simulink model "Alpha_Drone_Model"  (R2020b)
settings: Solver=VariableStepAuto  StartTime=0.0  StopTime=5  RelTol=1e-3
model workspace (MATLAB code in the model file):
  smiData = struct
  smiData.RigidTransform = struct
  smiData.Solid = struct
  smiData.PlanarJoint = struct
  smiData.PlanarJoint.Rz = struct
  smiData.PlanarJoint.Rz.Pos = -154.16759191545947
  smiData.PlanarJoint.Px = struct
  smiData.PlanarJoint.Px.Pos = 0
  smiData.PlanarJoint.Py = struct
  smiData.PlanarJoint.Py.Pos = 0
  smiData.PlanarJoint.ID = '[drone_pillar_test_2-1:-:drone_top_test_3-1]'
  smiData.PrismaticJoint = struct
  smiData.RevoluteJoint = struct
  other statements: smiData.RigidTransform(1).translation =    [0 0 0];; smiData.RigidTransform(1).angle = 3.1415926535897931;; smiData.RigidTransform(1).axis = [1 0 0];; smiData.RigidTransform(1).ID = ['B[drone_base_test_3-1:-:drone_camera_w'                                  'all_test-1]']; smiData.RigidTransform(2).translation =    [88.000000000000028 19.999999999999986 6.00000000000003];; smiData.RigidTransform(2).angle = 2.0943951023931953;; smiData.RigidTransform(2).axis = [0.57735026918962584 0.57735026918962584                                    -0.57735026; smiData.RigidTransform(2).ID = ['F[drone_base_test_3-1:-:drone_camera_w'                                  'all_test-1]']; smiData.RigidTransform(3).translation =    [0 0 0];; smiData.RigidTransform(3).angle = 3.1415926535897931;; smiData.RigidTransform(3).axis = [1 0 0];; smiData.RigidTransform(3).ID = ['B[drone_base_test_3-1:-:drone_camera_w'                                  'all_test-2]'] ... (+385)
undefined symbols (not defined in the file or in its folder): g, R, V1_trim, V3_trim, X, Y, Z
libraries: sm_lib x149, fl_lib x113, nesl_utility x52, ee_lib x16
(part 2 of 5)

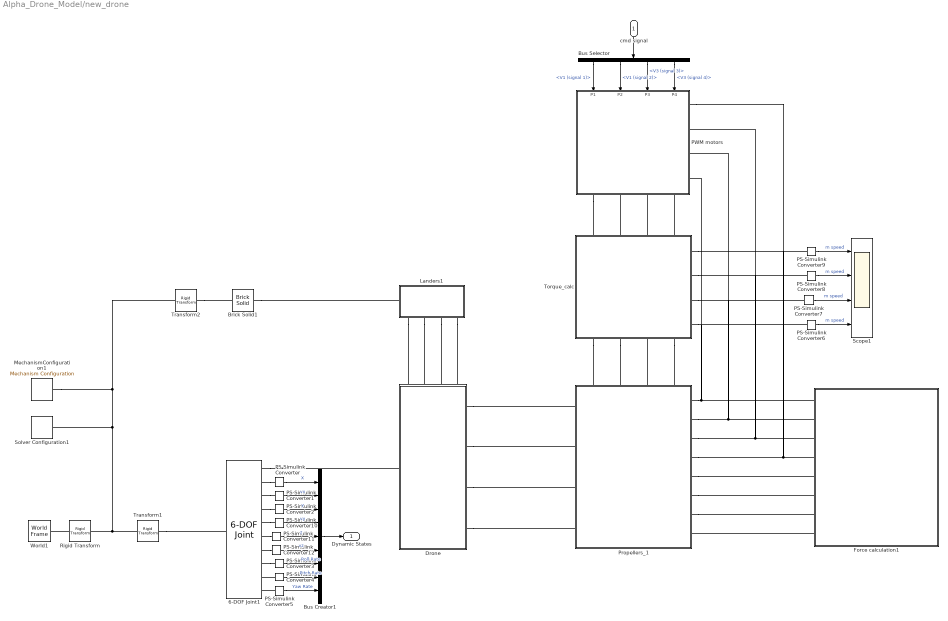
== system Alpha_Drone_Model/new_drone ==
  cmd signal : Inport
  6-DOF Joint1 : sm_lib/Joints/6-DOF Joint  JointMode=Normal  SenseConstraintForce=off  SenseConstraintForceX=off  SenseConstraintForceY=off  SenseConstraintForceZ=off  SenseConstraintTorque=off  SenseConstraintTorqueX=off  SenseConstraintTorqueY=off  SenseConstraintTorqueZ=off  SenseTotalForce=off  SenseTotalForceX=off  SenseTotalForceY=off  SenseTotalForceZ=off  SenseTotalTorque=off  SenseTotalTorqueX=off  SenseTotalTorqueY=off  SenseTotalTorqueZ=off  CompositeWrenchDir=FollowerOnBase  CompositeWrenchFrame=BaseFrame  PxEquilibriumPosition=0  PxEquilibriumPositionUnits=m  PxSpringStiffness=0  PxSpringStiffnessUnits=N/m  PxDampingCoefficient=air_damping  PxDampingCoefficientUnits=N/(m/s)  PxTorqueActuationMode=NoTorque  PxMotionActuationMode=ComputedMotion  PxSensePosition=on  PxSenseVelocity=on  PxSenseAcceleration=off  PxSenseTorqueForce=off  PxSenseLowerLimitTorqueForce=off  PxSenseUpperLimitTorqueForce=off  PxLowerLimitSpecify=off  PxLowerLimitBound=-1  PxLowerLimitBoundUnits=m  PxLowerLimitStiffness=1e6  PxLowerLimitStiffnessUnits=N/m  PxLowerLimitDamping=1e3  PxLowerLimitDampingUnits=N/(m/s)  PxLowerLimitTransitionRegionWidth=1e-4  PxLowerLimitTransitionRegionWidthUnits=m  PxUpperLimitSpecify=off  PxUpperLimitBound=1  PxUpperLimitBoundUnits=m  PxUpperLimitStiffness=1e6  PxUpperLimitStiffnessUnits=N/m  PxUpperLimitDamping=1e3  PxUpperLimitDampingUnits=N/(m/s)  PxUpperLimitTransitionRegionWidth=1e-4  PxUpperLimitTransitionRegionWidthUnits=m  PxPositionTargetSpecify=off  PxPositionTargetPriority=High  PxPositionTargetValue=0  PxPositionTargetValueUnits=m  PxVelocityTargetSpecify=off  PxVelocityTargetPriority=High  PxVelocityTargetValue=0  PxVelocityTargetValueUnits=m/s  PyEquilibriumPosition=0  PyEquilibriumPositionUnits=m  PySpringStiffness=0  PySpringStiffnessUnits=N/m  PyDampingCoefficient=air_damping  PyDampingCoefficientUnits=N/(m/s)  PyTorqueActuationMode=NoTorque  PyMotionActuationMode=ComputedMotion  PySensePosition=on  PySenseVelocity=on  PySenseAcceleration=off  PySenseTorqueForce=off  PySenseLowerLimitTorqueForce=off  PySenseUpperLimitTorqueForce=off  PyLowerLimitSpecify=off  PyLowerLimitBound=0  PyLowerLimitBoundUnits=m  PyLowerLimitStiffness=1e6  PyLowerLimitStiffnessUnits=N/m  PyLowerLimitDamping=1  PyLowerLimitDampingUnits=N/(m/s)  PyLowerLimitTransitionRegionWidth=1e4  PyLowerLimitTransitionRegionWidthUnits=m  PyUpperLimitSpecify=off  PyUpperLimitBound=1  PyUpperLimitBoundUnits=m  PyUpperLimitStiffness=1e6  PyUpperLimitStiffnessUnits=N/m  PyUpperLimitDamping=1e3  PyUpperLimitDampingUnits=N/(m/s)  PyUpperLimitTransitionRegionWidth=1e-4  PyUpperLimitTransitionRegionWidthUnits=m  PyPositionTargetSpecify=off  PyPositionTargetPriority=High  PyPositionTargetValue=0  PyPositionTargetValueUnits=m  PyVelocityTargetSpecify=off  PyVelocityTargetPriority=High  PyVelocityTargetValue=0  PyVelocityTargetValueUnits=m/s  PzEquilibriumPosition=0  PzEquilibriumPositionUnits=m  PzSpringStiffness=0  PzSpringStiffnessUnits=N/m  PzDampingCoefficient=air_damping  PzDampingCoefficientUnits=N/(m/s)  PzTorqueActuationMode=NoTorque  PzMotionActuationMode=ComputedMotion  PzSensePosition=on  PzSenseVelocity=on  PzSenseAcceleration=off  PzSenseTorqueForce=off  PzSenseLowerLimitTorqueForce=off  PzSenseUpperLimitTorqueForce=off  PzLowerLimitSpecify=off  PzLowerLimitBound=-1  PzLowerLimitBoundUnits=m  PzLowerLimitStiffness=1e6  PzLowerLimitStiffnessUnits=N/m  PzLowerLimitDamping=1e3  PzLowerLimitDampingUnits=N/(m/s)  PzLowerLimitTransitionRegionWidth=1e-4  PzLowerLimitTransitionRegionWidthUnits=m  PzUpperLimitSpecify=off  PzUpperLimitBound=1  PzUpperLimitBoundUnits=m  PzUpperLimitStiffness=1e6  PzUpperLimitStiffnessUnits=N/m  PzUpperLimitDamping=1e3  PzUpperLimitDampingUnits=N/(m/s)  PzUpperLimitTransitionRegionWidth=1e-4  PzUpperLimitTransitionRegionWidthUnits=m  PzPositionTargetSpecify=off  PzPositionTargetPriority=High  PzPositionTargetValue=0  PzPositionTargetValueUnits=m  PzVelocityTargetSpecify=off  PzVelocityTargetPriority=High  PzVelocityTargetValue=0  PzVelocityTargetValueUnits=m/s  SphDefPosRotationMethod=None  SphDefPosRotationAngleUnits=deg  SphDefPosRotationStandardAxis=+Z  SphDefPosRotationAngle=0.0  SphDefPosRotationArbitraryAxis=[0 0 1]  SphDefPosFollAlignAxisA=+X  SphDefPosBaseAlignAxisA=+Y  SphDefPosFollAlignAxisB=+Y  SphDefPosBaseAlignAxisB=+Z  SphDefPosRotationSequenceAxes=FollowerAxes  SphDefPosRotationSequence=XYX  SphDefPosRotationSequenceAngles=[0 0 0]  SphDefPosRotationSequenceAnglesUnits=deg  SphDefPosRotationMatrix=[1 0 0; 0 1 0; 0 0 1]  SphEqPosRotationMethod=None  SphEqPosRotationAngleUnits=deg  SphEqPosRotationStandardAxis=+Z  SphEqPosRotationAngle=0.0  SphEqPosRotationArbitraryAxis=[0 0 1]  SphEqPosFollAlignAxisA=+X  SphEqPosBaseAlignAxisA=+Y  SphEqPosFollAlignAxisB=+Y  SphEqPosBaseAlignAxisB=+Z  SphEqPosRotationSequenceAxes=FollowerAxes  SphEqPosRotationSequence=XYX  SphEqPosRotationSequenceAngles=[0 0 0]  SphEqPosRotationSequenceAnglesUnits=deg  SphEqPosRotationMatrix=[1 0 0; 0 1 0; 0 0 1]  SphSpringStiffness=0  SphSpringStiffnessUnits=N*m/deg  SphDampingCoefficient=air_damping  SphDampingCoefficientUnits=N*m/(deg/s)  SphActuateTorqueX=off  SphActuateTorqueY=off  SphActuateTorqueZ=off  SphActuateTorque=off  SphTorqueActuationMode=NoTorque  SphMotionActuationMode=ComputedMotion  SphActuationFrame=BaseFrame  SphSensePosition=off  SphSenseVelocityX=on  SphSenseVelocityY=on  SphSenseVelocityZ=on  SphSenseVelocity=off  SphSenseAccelerationX=off  SphSenseAccelerationY=off  SphSenseAccelerationZ=off  SphSenseAcceleration=off  SphSenseTorqueX=off  SphSenseTorqueY=off  SphSenseTorqueZ=off  SphSenseTorqueForce=off  SphSenseLowerLimitTorqueMag=off  SphSenseUpperLimitTorqueMag=off  SphSensingFrame=BaseFrame  SphLowerLimitSpecify=off  SphLowerLimitBound=15  SphLowerLimitBoundUnits=deg  SphLowerLimitStiffness=1e4  SphLowerLimitStiffnessUnits=N*m/deg  SphLowerLimitDamping=10  SphLowerLimitDampingUnits=N*m/(deg/s)  SphLowerLimitTransitionRegionWidth=0.1  SphLowerLimitTransitionRegionWidthUnits=deg  SphUpperLimitSpecify=off  SphUpperLimitBound=45  SphUpperLimitBoundUnits=deg  SphUpperLimitStiffness=1e4  SphUpperLimitStiffnessUnits=N*m/deg  SphUpperLimitDamping=10  SphUpperLimitDampingUnits=N*m/(deg/s)  SphUpperLimitTransitionRegionWidth=0.1  SphUpperLimitTransitionRegionWidthUnits=deg  SphPositionTargetRotationMethod=AlignedAxes  SphPositionTargetRotationAngleUnits=deg  SphPositionTargetRotationStandardAxis=+Z  SphPositionTargetRotationAngle=0.0  SphPositionTargetRotationArbitraryAxis=[0 0 1]  SphPositionTargetFollAlignAxisA=+X  SphPositionTargetBaseAlignAxisA=+X  SphPositionTargetFollAlignAxisB=+Y  SphPositionTargetBaseAlignAxisB=+Y  SphPositionTargetRotationSequenceAxes=FollowerAxes  SphPositionTargetRotationSequence=XYX  SphPositionTargetRotationSequenceAngles=[0 0 0]  SphPositionTargetRotationSequenceAnglesUnits=deg  SphPositionTargetRotationMatrix=[1 0 0; 0 1 0; 0 0 1]  SphPositionTargetSpecify=off  SphPositionTargetPriority=High  SphVelocityTargetValue=[0 0 0]  SphVelocityTargetValueUnits=deg/s  SphVelocityTargetSpecify=off  SphVelocityTargetPriority=High  SphVelocityTargetInFollowerFrame=on
  Brick Solid1 : sm_lib/Body Elements/Brick Solid  GraphicAmbientColor=[0.15 0.15 0.15 1.0]  BasedOnType=Density  BrickDimensions=[1 1 0.1]  BrickDimensionUnits=m  CenterOfMass=[0 0 0]  CenterOfMassUnits=m  GraphicDiffuseColor=[0.0 0.6 0.2]  Density=1000  DensityUnits=kg/m^3  DoExposeReferenceFrame=on  GraphicEmissiveColor=[0.0 0.0 0.0 1.0]  ExportEntireGeometry=on  SerializedFrames=<Frames/>  MarkerShape=Sphere  MarkerSize=10  GraphicType=FromGeometry  InertiaType=CalculateFromGeometry  Mass=1  MassUnits=kg  MomentsOfInertia=[1 1 1]  MomentsOfInertiaUnits=kg*m^2  GraphicOpacity=1.0  ProductsOfInertia=[0 0 0]  ProductsOfInertiaUnits=kg*m^2  GraphicShininess=75  GraphicSpecularColor=[0.5 0.5 0.5 1.0]  GraphicVisPropType=SimpleVisualProperties
  Bus Creator1 : BusCreator  Inputs=9
  Bus Selector : BusSelector  OutputSignals=V1 (signal 1),V1 (signal 2),V3 (signal 3),V3 (signal 4)
  Drone : Subsystem
      settings: PortSchema="{\"entries\":[{\"content\":{\"sides\":[{\"content\":{\"connectorIds\":[\"LConn1\"]},\"type\":\"ConnectorPlacement.EquallySpacedRectSide\",\"uuid\":\"2ddff43e-b9b9-4f8b-b52c-32ef76abc7f2\"},{\"content\":{\"connectorIds\":[\"RConn1\",\"RConn2\",\"RConn3\",\"RConn4\"],\"side\":\"RIGHT\"},\"type\":\"ConnectorPlacement.EquallySpacedRectSide\",\"uuid\":\"84cdcda4-30ad-4435-863c-4e05e54e1cee\"},{\"content\":{\"connectorIds\":[\"LConn2\",\"LConn3\",\"LConn4\",\"LConn5\"],\"side\":\"TOP\"},\"type\":\"ConnectorPlacement.EquallySpacedRectSide\",\"uuid\":\"12774c4c-303b-498f-8577-32bcc0aee797\"},{\"content\":{\"connectorIds\":[],\"side\":\"HIDDEN\"},\"type\":\"ConnectorPlacement.EquallySpacedRectSide\",\"uuid\":\"2c89ce61-ca11-462f-b06b-bd195c97151b\"}]},\"type\":\"ConnectorPlacement.EquallySpacedConnector\",\"uuid\":\"ae66c99c-2a8a-4601-9c2b-027ea84a534a\"}],\"packageUris\":[\"http://schema.mathworks.com/mf0/Connector/R2020b\"],\"version\":\"1.0\"}"
  Force calculation1 : Subsystem
  Landers1 : Subsystem
      settings: PortSchema="{\"entries\":[{\"content\":{\"sides\":[{\"content\":{\"connectorIds\":[]},\"type\":\"ConnectorPlacement.EquallySpacedRectSide\",\"uuid\":\"29ed25fe-b3f0-40d8-8e38-dad31f47c1c2\"},{\"content\":{\"connectorIds\":[\"RConn1\"],\"side\":\"RIGHT\"},\"type\":\"ConnectorPlacement.EquallySpacedRectSide\",\"uuid\":\"a44326be-c514-4699-a20f-f031abb9163a\"},{\"content\":{\"connectorIds\":[\"LConn1\",\"LConn2\",\"LConn3\",\"LConn4\"],\"side\":\"TOP\"},\"type\":\"ConnectorPlacement.EquallySpacedRectSide\",\"uuid\":\"e989b3f4-324c-4714-b27e-b8d073d4c35f\"},{\"content\":{\"connectorIds\":[],\"side\":\"HIDDEN\"},\"type\":\"ConnectorPlacement.EquallySpacedRectSide\",\"uuid\":\"003ab62d-37b6-4b48-957b-1f2b95d598b0\"}]},\"type\":\"ConnectorPlacement.EquallySpacedConnector\",\"uuid\":\"ee59c263-ccee-4526-9944-481878d464b1\"}],\"packageUris\":[\"http://schema.mathworks.com/mf0/Connector/R2020b\"],\"version\":\"1.0\"}"
  MechanismConfiguration1 : sm_lib/Utilities/Mechanism Configuration  UniformGravity=Constant  GravityVector=[0 0 g]  GravityVectorUnits=m/s^2  GravityUnits=m/s^2  LinearizationDelta=0.001  JointModeTransitionNonlinearIterations=2
  PS-Simulink Converter{,1..5,10..12} (9 alike) : nesl_utility/PS-Simulink Converter  PhysicalDomain=network_engine_domain  SubClassName=ps_output  LeftPortType=input  RightPortType=output  PseudoPeriodic=off  Frequencies=[]  Unit=inherit  AffineConversion=off
  PS-Simulink Converter{6..9} (4 alike) : nesl_utility/PS-Simulink Converter  PhysicalDomain=network_engine_domain  SubClassName=ps_output  LeftPortType=input  RightPortType=output  PseudoPeriodic=off  Frequencies=[]  Unit=rpm  AffineConversion=off
  PWM motors : Subsystem
      settings: PortSchema="{\"entries\":[{\"content\":{\"sides\":[{\"content\":{\"connectorIds\":[\"In1\",\"In2\",\"In3\",\"In4\"]},\"type\":\"ConnectorPlacement.EquallySpacedRectSide\",\"uuid\":\"0aa47eaa-b314-49af-ba20-9f866096b1c7\"},{\"content\":{\"connectorIds\":[\"RConn1\",\"RConn2\",\"RConn3\",\"RConn4\"],\"side\":\"RIGHT\"},\"type\":\"ConnectorPlacement.EquallySpacedRectSide\",\"uuid\":\"be00fcf1-f0c0-4679-a976-81a7113ef2f3\"},{\"content\":{\"connectorIds\":[],\"side\":\"TOP\"},\"type\":\"ConnectorPlacement.EquallySpacedRectSide\",\"uuid\":\"744c4fca-265d-4f23-9ed8-a5ce9174507b\"},{\"content\":{\"connectorIds\":[\"RConn5\",\"RConn6\",\"RConn7\",\"RConn8\"],\"side\":\"BOTTOM\"},\"type\":\"ConnectorPlacement.EquallySpacedRectSide\",\"uuid\":\"b07c2b3a-f3e9-41e5-9730-85c6be094db7\"},{\"content\":{\"connectorIds\":[],\"side\":\"HIDDEN\"},\"type\":\"ConnectorPlacement.EquallySpacedRectSide\",\"uuid\":\"b49dea78-7ad3-4d52-b3a6-72cc1bd77d5e\"}]},\"type\":\"ConnectorPlacement.EquallySpacedConnector\",\"uuid\":\"57264236-7f66-4868-aca9-e0c74f83ab49\"}],\"packageUris\":[\"http://schema.mathworks.com/mf0/Connector/R2020b\"],\"version\":\"1.0\"}"
  Propellers_1 : Subsystem
      settings: PortSchema="{\"entries\":[{\"content\":{\"sides\":[{\"content\":{\"connectorIds\":[\"LConn1\",\"LConn2\",\"LConn3\",\"LConn4\"]},\"type\":\"ConnectorPlacement.EquallySpacedRectSide\",\"uuid\":\"b250e274-2fd6-45d7-b915-b466c5f9d255\"},{\"content\":{\"connectorIds\":[\"RConn1\",\"RConn2\",\"RConn3\",\"RConn4\",\"RConn5\",\"RConn6\",\"RConn7\",\"RConn8\"],\"side\":\"RIGHT\"},\"type\":\"ConnectorPlacement.EquallySpacedRectSide\",\"uuid\":\"c76b79cf-ecc8-43fa-b8c8-dc402773d11f\"},{\"content\":{\"connectorIds\":[\"LConn5\",\"LConn6\",\"LConn7\",\"LConn8\"],\"side\":\"TOP\"},\"type\":\"ConnectorPlacement.EquallySpacedRectSide\",\"uuid\":\"3950bb13-7450-4adc-a891-c6053fed2cc6\"},{\"content\":{\"connectorIds\":[],\"side\":\"HIDDEN\"},\"type\":\"ConnectorPlacement.EquallySpacedRectSide\",\"uuid\":\"c1ecd3aa-adb0-4a11-9d33-da842965230c\"}]},\"type\":\"ConnectorPlacement.EquallySpacedConnector\",\"uuid\":\"e31fcf3f-0f5a-48dc-bc44-b2ff7b3cb046\"}],\"packageUris\":[\"http://schema.mathworks.com/mf0/Connector/R2020b\"],\"version\":\"1.0\"}"
  Rigid Transform : sm_lib/Frames and Transforms/Rigid Transform  TranslationMethod=None  TranslationStandardOffset=0  TranslationLengthUnit=m  TranslationStandardAxis=+Z  TranslationCartesianOffset=[0 0 0]  TranslationROffset=0  TranslationROffsetUnits=m  TranslationZOffset=0  TranslationZOffsetUnits=m  TranslationThetaOffset=0  TranslationThetaOffsetUnits=deg  RotationMethod=StandardAxis  RotationAngleUnits=deg  RotationStandardAxis=+X  RotationAngle=180  RotationArbitraryAxis=[0 0 1]  FollAlignAxisA=+X  BaseAlignAxisA=+Y  FollAlignAxisB=+Y  BaseAlignAxisB=+Z  RotationSequenceAxes=FollowerAxes  RotationSequence=XYX  RotationSequenceAngles=[0 0 0]  RotationSequenceAnglesUnits=deg  RotationMatrix=[1 0 0; 0 1 0; 0 0 1]
  Scope1 : Scope  NumInputPorts=4
  Solver Configuration1 : nesl_utility/Solver Configuration  PhysicalDomain=network_engine_domain  SubClassName=solver  LeftPortType=input  RightPortType=generic  Tones=[]  Harmonics=[]  SimulateNoise=off  Profile=off  UseLocalSampling=off  EnableSwitchedLinearOptims=on  FrequencyDomain=off  UseCCode=off  RelTol=0.001  AbsTol=1e-06  MinStep=1e-09  ToWorkspace=off  RevertToSquareIcSolve=off  NumHomotopyIterations=100  PhasorMode=off  PhasorModeNumHarmonics=1  DoDC=off  ResidualTolerance=1e-09  UseLocalSolver=off  LocalSolverChoice=NE_BACKWARD_EULER_ADVANCER  LocalSolverSampleTime=0.001  DoFixedCost=off  MaxNonlinIter=3  MaxModeIter=2  ComputeImpulses=off  ImpulseIterations=2  LinearAlgebra=auto  EquationFormulation=NE_TIME_EF  DelaysMemoryBudget=1024  AutomaticFiltering=on  FilteringTimeConstant=0.001  PartitionStorageMethod=AS_NEEDED  PartitionMemoryBudget=1024  PartitionMethod=ROBUST
  Torque_calc : Subsystem
      settings: PortSchema="{\"entries\":[{\"content\":{\"sides\":[{\"content\":{\"connectorIds\":[]},\"type\":\"ConnectorPlacement.EquallySpacedRectSide\",\"uuid\":\"eea3dfa4-6c4f-447d-9f2a-f18a83183d98\"},{\"content\":{\"connectorIds\":[\"RConn1\",\"RConn2\",\"RConn3\",\"RConn4\"],\"side\":\"RIGHT\"},\"type\":\"ConnectorPlacement.EquallySpacedRectSide\",\"uuid\":\"c604e34d-0590-453f-bf6c-420895a89f4d\"},{\"content\":{\"connectorIds\":[\"LConn1\",\"LConn2\",\"LConn3\",\"LConn4\"],\"side\":\"TOP\"},\"type\":\"ConnectorPlacement.EquallySpacedRectSide\",\"uuid\":\"50bcecdb-52f6-4b25-bece-8e6a846b7dd0\"},{\"content\":{\"connectorIds\":[\"RConn5\",\"RConn6\",\"RConn7\",\"RConn8\"],\"side\":\"BOTTOM\"},\"type\":\"ConnectorPlacement.EquallySpacedRectSide\",\"uuid\":\"c913db90-ccc2-4f4f-a5da-6c9411a23c28\"},{\"content\":{\"connectorIds\":[],\"side\":\"HIDDEN\"},\"type\":\"ConnectorPlacement.EquallySpacedRectSide\",\"uuid\":\"0f1aeb6e-b451-4600-ac15-69882e2b4329\"}]},\"type\":\"ConnectorPlacement.EquallySpacedConnector\",\"uuid\":\"f9536a7f-9aaa-4e3e-af48-cb10a5d231a4\"}],\"packageUris\":[\"http://schema.mathworks.com/mf0/Connector/R2020b\"],\"version\":\"1.0\"}"
  Transform1 : sm_lib/Frames and Transforms/Rigid Transform  TranslationMethod=StandardAxis  TranslationStandardOffset=0.1  TranslationLengthUnit=m  TranslationStandardAxis=-Z  TranslationCartesianOffset=smiData.RigidTransform(63).translation  TranslationROffset=0  TranslationROffsetUnits=m  TranslationZOffset=0  TranslationZOffsetUnits=m  TranslationThetaOffset=0  TranslationThetaOffsetUnits=deg  RotationMethod=None  RotationAngleUnits=rad  RotationStandardAxis=+Z  RotationAngle=smiData.RigidTransform(63).angle  RotationArbitraryAxis=smiData.RigidTransform(63).axis  FollAlignAxisA=+X  BaseAlignAxisA=+Y  FollAlignAxisB=+Y  BaseAlignAxisB=+Z  RotationSequenceAxes=FollowerAxes  RotationSequence=XYX  RotationSequenceAngles=[0 0 0]  RotationSequenceAnglesUnits=deg  RotationMatrix=[1 0 0; 0 1 0; 0 0 1]
  Transform2 : sm_lib/Frames and Transforms/Rigid Transform  TranslationMethod=StandardAxis  TranslationStandardOffset=0.05  TranslationLengthUnit=m  TranslationStandardAxis=+Z  TranslationCartesianOffset=smiData.RigidTransform(63).translation  TranslationROffset=0  TranslationROffsetUnits=m  TranslationZOffset=0  TranslationZOffsetUnits=m  TranslationThetaOffset=0  TranslationThetaOffsetUnits=deg  RotationMethod=None  RotationAngleUnits=deg  RotationStandardAxis=+X  RotationAngle=180  RotationArbitraryAxis=smiData.RigidTransform(63).axis  FollAlignAxisA=+X  BaseAlignAxisA=+Y  FollAlignAxisB=+Y  BaseAlignAxisB=+Z  RotationSequenceAxes=FollowerAxes  RotationSequence=XYX  RotationSequenceAngles=[0 0 0]  RotationSequenceAnglesUnits=deg  RotationMatrix=[1 0 0; 0 1 0; 0 0 1]
  World1 : sm_lib/Frames and Transforms/World Frame
  Dynamic States : Outport
  wires:
  PS-Simulink Converter4/1 -> Bus Creator1/8  "Pitch Rate"
  PS-Simulink Converter/1 -> Bus Creator1/1  "X"
  PS-Simulink Converter3/1 -> Bus Creator1/7  "Roll Rate"
  PS-Simulink Converter5/1 -> Bus Creator1/9  "Yaw Rate"
  Bus Creator1/1 -> Dynamic States/1
  PS-Simulink Converter6/1 -> Scope1/4  "m speed"
  PS-Simulink Converter7/1 -> Scope1/3  "m speed"
  PS-Simulink Converter8/1 -> Scope1/2  "m speed"
  PS-Simulink Converter9/1 -> Scope1/1  "m speed"
  cmd signal/1 -> Bus Selector/1
  PS-Simulink Converter2/1 -> Bus Creator1/3  "y"
  PS-Simulink Converter11/1 -> Bus Creator1/5  "z"
  PS-Simulink Converter1/1 -> Bus Creator1/2  "vx"
  PS-Simulink Converter10/1 -> Bus Creator1/4  "vy"
  PS-Simulink Converter12/1 -> Bus Creator1/6  "vz"
  Bus Selector/1 -> PWM motors/1(P1)  "<V1 (signal 1)>"
  Bus Selector/2 -> PWM motors/2(P2)  "<V1 (signal 2)>"
  Bus Selector/3 -> PWM motors/3(P3)  "<V3 (signal 3)>"
  Bus Selector/4 -> PWM motors/4(P4)  "<V3 (signal 4)>"
  connections:
  Propellers_1/RConn1 -- PS-Simulink Converter6/LConn1 -- Torque_calc/RConn4 -- PWM motors/RConn8 -- Force calculation1/LConn1
  Landers1/LConn1 -- Drone/LConn5
  Propellers_1/RConn7 -- Force calculation1/LConn7
  Propellers_1/RConn4 -- PWM motors/RConn5 -- PS-Simulink Converter9/LConn1 -- Torque_calc/RConn1 -- Force calculation1/LConn4
  Landers1/LConn2 -- Drone/LConn4
  Drone/RConn1 -- Propellers_1/LConn1
  Landers1/LConn4 -- Drone/LConn2
  Propellers_1/RConn6 -- Force calculation1/LConn6
  Propellers_1/RConn5 -- Force calculation1/LConn5
  Drone/RConn4 -- Propellers_1/LConn4
  Landers1/LConn3 -- Drone/LConn3
  Drone/RConn3 -- Propellers_1/LConn3
  Force calculation1/LConn8 -- Propellers_1/RConn8
  Drone/RConn2 -- Propellers_1/LConn2
  Propellers_1/RConn3 -- PS-Simulink Converter8/LConn1 -- Torque_calc/RConn2 -- PWM motors/RConn6 -- Force calculation1/LConn3
  Propellers_1/RConn2 -- Force calculation1/LConn2 -- PWM motors/RConn7 -- PS-Simulink Converter7/LConn1 -- Torque_calc/RConn3
  PWM motors/RConn1 -- Torque_calc/LConn1
  Torque_calc/LConn3 -- PWM motors/RConn3
  Torque_calc/LConn2 -- PWM motors/RConn2
  Torque_calc/LConn4 -- PWM motors/RConn4
  Torque_calc/RConn5 -- Propellers_1/LConn5
  Propellers_1/LConn7 -- Torque_calc/RConn7
  Torque_calc/RConn6 -- Propellers_1/LConn6
  Torque_calc/RConn8 -- Propellers_1/LConn8
  Transform2/RConn1 -- Brick Solid1/RConn1
  Transform1/LConn1 -- Rigid Transform/RConn1 -- Transform2/LConn1 -- MechanismConfiguration1/RConn1 -- Solver Configuration1/RConn1
  Brick Solid1/LConn1 -- Landers1/RConn1
  Rigid Transform/LConn1 -- World1/RConn1
  6-DOF Joint1/RConn8 -- PS-Simulink Converter3/LConn1
  PS-Simulink Converter4/LConn1 -- 6-DOF Joint1/RConn9
  PS-Simulink Converter5/LConn1 -- 6-DOF Joint1/RConn10
  6-DOF Joint1/RConn2 -- PS-Simulink Converter/LConn1
  6-DOF Joint1/RConn3 -- PS-Simulink Converter1/LConn1
  6-DOF Joint1/RConn4 -- PS-Simulink Converter2/LConn1
  6-DOF Joint1/RConn5 -- PS-Simulink Converter10/LConn1
  6-DOF Joint1/RConn6 -- PS-Simulink Converter11/LConn1
  6-DOF Joint1/RConn7 -- PS-Simulink Converter12/LConn1
  Transform1/RConn1 -- 6-DOF Joint1/LConn1
  6-DOF Joint1/RConn1 -- Drone/LConn1

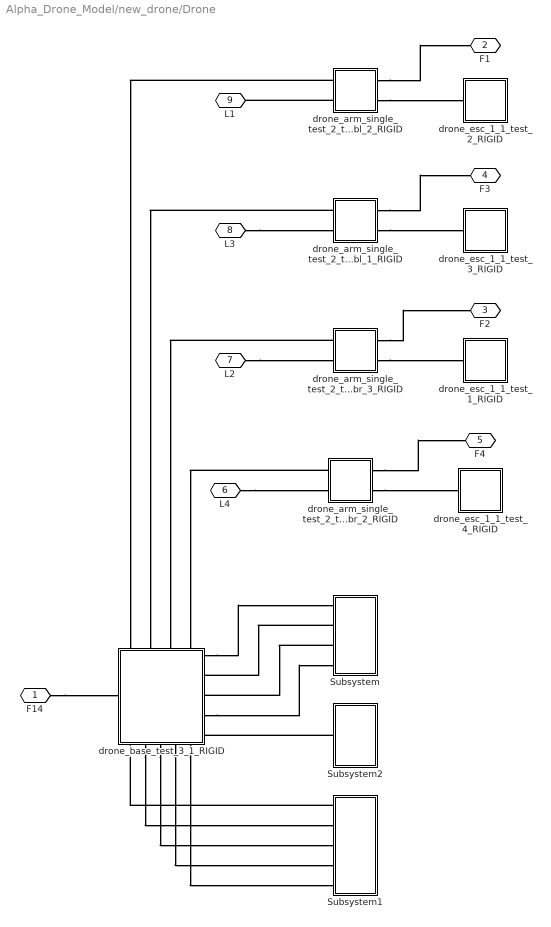
== system Alpha_Drone_Model/new_drone/Drone ==
  Subsystem : Subsystem
  Subsystem1 : Subsystem
  Subsystem2 : Subsystem
  drone_arm_single_test_2_tl_br_2_RIGID : Subsystem
  drone_arm_single_test_2_tl_br_3_RIGID : Subsystem
  drone_arm_single_test_2_tr_bl_1_RIGID : Subsystem
  drone_arm_single_test_2_tr_bl_2_RIGID : Subsystem
  drone_base_test_3_1_RIGID : Subsystem
      settings: PortSchema="{\"entries\":[{\"content\":{\"sides\":[{\"content\":{\"connectorIds\":[\"LConn1\"]},\"type\":\"ConnectorPlacement.EquallySpacedRectSide\",\"uuid\":\"3979f689-f2e7-42c3-80af-f898cffc6627\"},{\"content\":{\"connectorIds\":[\"RConn1\",\"RConn2\",\"RConn3\",\"RConn4\",\"RConn5\"],\"side\":\"RIGHT\"},\"type\":\"ConnectorPlacement.EquallySpacedRectSide\",\"uuid\":\"d5df15a2-0509-4ce9-a78a-c9b521a28f2c\"},{\"content\":{\"connectorIds\":[\"LConn2\",\"LConn3\",\"LConn4\",\"LConn5\"],\"side\":\"TOP\"},\"type\":\"ConnectorPlacement.EquallySpacedRectSide\",\"uuid\":\"a062ce0d-f5a1-4bb9-aa4f-f81fc5481e55\"},{\"content\":{\"connectorIds\":[\"RConn6\",\"RConn7\",\"RConn8\",\"RConn9\",\"RConn10\"],\"side\":\"BOTTOM\"},\"type\":\"ConnectorPlacement.EquallySpacedRectSide\",\"uuid\":\"9e3fb357-542a-46da-bf60-66e0768f6863\"},{\"content\":{\"connectorIds\":[],\"side\":\"HIDDEN\"},\"type\":\"ConnectorPlacement.EquallySpacedRectSide\",\"uuid\":\"788c0c2e-9632-4521-be72-6a644cdbf0ea\"}]},\"type\":\"ConnectorPlacement.EquallySpacedConnector\",\"uuid\":\"1be13487-ca5d-4f55-9a83-a878693f11fe\"}],\"packageUris\":[\"http://schema.mathworks.com/mf0/Connector/R2020b\"],\"version\":\"1.0\"}"
  drone_esc_1_1_test_1_RIGID : Subsystem
  drone_esc_1_1_test_2_RIGID : Subsystem
  drone_esc_1_1_test_3_RIGID : Subsystem
  drone_esc_1_1_test_4_RIGID : Subsystem
  F14 : PMIOPort  Side=Left
  F1 : PMIOPort  Port=2  Side=Right
  F2 : PMIOPort  Port=3  Side=Right
  F3 : PMIOPort  Port=4  Side=Right
  F4 : PMIOPort  Port=5  Side=Right
  L4 : PMIOPort  Port=6  Side=Left
  L2 : PMIOPort  Port=7  Side=Left
  L3 : PMIOPort  Port=8  Side=Left
  L1 : PMIOPort  Port=9  Side=Left
  connections:
  drone_arm_single_test_2_tr_bl_1_RIGID/RConn2 -- drone_esc_1_1_test_3_RIGID/LConn1
  drone_arm_single_test_2_tr_bl_2_RIGID/LConn1 -- drone_base_test_3_1_RIGID/LConn2
  drone_arm_single_test_2_tr_bl_1_RIGID/RConn1 -- F3/RConn1
  drone_arm_single_test_2_tl_br_2_RIGID/RConn2 -- drone_esc_1_1_test_4_RIGID/LConn1
  drone_arm_single_test_2_tl_br_2_RIGID/RConn1 -- F4/RConn1
  drone_arm_single_test_2_tl_br_3_RIGID/RConn2 -- drone_esc_1_1_test_1_RIGID/LConn1
  drone_arm_single_test_2_tr_bl_2_RIGID/RConn2 -- drone_esc_1_1_test_2_RIGID/LConn1
  F14/RConn1 -- drone_base_test_3_1_RIGID/LConn1
  drone_arm_single_test_2_tr_bl_1_RIGID/LConn1 -- drone_base_test_3_1_RIGID/LConn3
  drone_arm_single_test_2_tl_br_2_RIGID/LConn1 -- drone_base_test_3_1_RIGID/LConn5
  drone_arm_single_test_2_tl_br_3_RIGID/LConn1 -- drone_base_test_3_1_RIGID/LConn4
  drone_arm_single_test_2_tr_bl_2_RIGID/RConn1 -- F1/RConn1
  drone_arm_single_test_2_tl_br_3_RIGID/RConn1 -- F2/RConn1
  drone_base_test_3_1_RIGID/RConn1 -- Subsystem/LConn1
  Subsystem/LConn2 -- drone_base_test_3_1_RIGID/RConn2
  Subsystem/LConn3 -- drone_base_test_3_1_RIGID/RConn3
  drone_base_test_3_1_RIGID/RConn4 -- Subsystem/LConn4
  drone_arm_single_test_2_tr_bl_2_RIGID/LConn2 -- L1/RConn1
  L3/RConn1 -- drone_arm_single_test_2_tr_bl_1_RIGID/LConn2
  L2/RConn1 -- drone_arm_single_test_2_tl_br_3_RIGID/LConn2
  L4/RConn1 -- drone_arm_single_test_2_tl_br_2_RIGID/LConn2
  Subsystem1/LConn1 -- drone_base_test_3_1_RIGID/RConn6
  drone_base_test_3_1_RIGID/RConn7 -- Subsystem1/LConn2
  drone_base_test_3_1_RIGID/RConn8 -- Subsystem1/LConn3
  drone_base_test_3_1_RIGID/RConn9 -- Subsystem1/LConn4
  drone_base_test_3_1_RIGID/RConn10 -- Subsystem1/LConn5
  Subsystem2/LConn1 -- drone_base_test_3_1_RIGID/RConn5

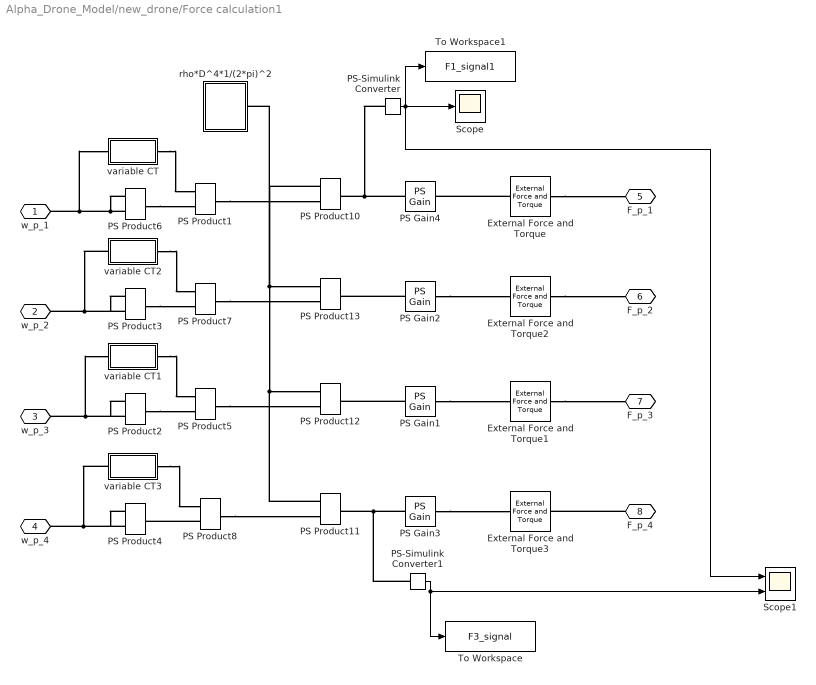
== system Alpha_Drone_Model/new_drone/Force calculation1 ==
  External Force and Torque{,1..3} (4 alike) : sm_lib/Forces and Torques/External Force and Torque  ForceResolutionFrame=AttachedFrame  EnableForceX=off  EnableForceY=off  EnableForceZ=on  EnableForce=off  TorqueResolutionFrame=AttachedFrame  EnableTorqueX=off  EnableTorqueY=off  EnableTorqueZ=off  EnableTorque=off
  PS Gain1 : fl_lib/Physical Signals/Functions/PS Gain  gain=1
  PS Gain2 : fl_lib/Physical Signals/Functions/PS Gain  gain=-1
  PS Gain3 : fl_lib/Physical Signals/Functions/PS Gain  gain=-1
  PS Gain4 : fl_lib/Physical Signals/Functions/PS Gain  gain=1
  PS Product{1..8,10..13} (12 alike) : fl_lib/Physical Signals/Functions/PS Product
  PS-Simulink Converter : nesl_utility/PS-Simulink Converter  PhysicalDomain=network_engine_domain  SubClassName=ps_output  LeftPortType=input  RightPortType=output  PseudoPeriodic=off  Frequencies=[]  Unit=inherit  AffineConversion=off
  PS-Simulink Converter1 : nesl_utility/PS-Simulink Converter  PhysicalDomain=network_engine_domain  SubClassName=ps_output  LeftPortType=input  RightPortType=output  PseudoPeriodic=off  Frequencies=[]  Unit=inherit  AffineConversion=off
  Scope : Scope
  Scope1 : Scope  NumInputPorts=2
  To Workspace : ToWorkspace  VariableName=F3_signal  SampleTime=-1
  To Workspace1 : ToWorkspace  VariableName=F1_signal1  SampleTime=-1
  rho*D^4*1/(2*pi)^2 : Subsystem
  variable CT : Subsystem
  variable CT1 : Subsystem
  variable CT2 : Subsystem
  variable CT3 : Subsystem
  w_p_1 : PMIOPort  Side=Left
  w_p_2 : PMIOPort  Port=2  Side=Left
  w_p_3 : PMIOPort  Port=3  Side=Left
  w_p_4 : PMIOPort  Port=4  Side=Left
  F_p_1 : PMIOPort  Port=5  Side=Left
  F_p_2 : PMIOPort  Port=6  Side=Left
  F_p_3 : PMIOPort  Port=7  Side=Left
  F_p_4 : PMIOPort  Port=8  Side=Left
  wires:
  PS-Simulink Converter/1 -> To Workspace1/1, Scope1/1, Scope/1
  PS-Simulink Converter1/1 -> To Workspace/1, Scope1/2
  connections:
  External Force and Torque2/RConn1 -- F_p_2/RConn1
  External Force and Torque/RConn1 -- F_p_1/RConn1
  External Force and Torque1/RConn1 -- F_p_3/RConn1
  F_p_4/RConn1 -- External Force and Torque3/RConn1
  PS Product6/LConn2 -- PS Product6/LConn1 -- w_p_1/RConn1 -- variable CT/LConn1
  External Force and Torque/LConn1 -- PS Gain4/RConn1
  PS Gain1/RConn1 -- External Force and Torque1/LConn1
  PS Gain2/RConn1 -- External Force and Torque2/LConn1
  PS Gain3/RConn1 -- External Force and Torque3/LConn1
  PS-Simulink Converter/LConn1 -- PS Product10/RConn1 -- PS Gain4/LConn1
  PS-Simulink Converter1/LConn1 -- PS Product11/RConn1 -- PS Gain3/LConn1
  PS Product2/LConn2 -- PS Product2/LConn1 -- variable CT1/LConn1 -- w_p_3/RConn1
  PS Product3/LConn2 -- PS Product3/LConn1 -- variable CT2/LConn1 -- w_p_2/RConn1
  PS Product4/LConn2 -- PS Product4/LConn1 -- variable CT3/LConn1 -- w_p_4/RConn1
  variable CT/RConn1 -- PS Product1/LConn1
  rho*D^4*1/(2*pi)^2/RConn1 -- PS Product10/LConn1 -- PS Product11/LConn1 -- PS Product12/LConn1 -- PS Product13/LConn1
  PS Product6/RConn1 -- PS Product1/LConn2
  PS Product1/RConn1 -- PS Product10/LConn2
  variable CT1/RConn1 -- PS Product5/LConn1
  PS Product2/RConn1 -- PS Product5/LConn2
  PS Product5/RConn1 -- PS Product12/LConn2
  PS Product3/RConn1 -- PS Product7/LConn2
  variable CT2/RConn1 -- PS Product7/LConn1
  PS Product7/RConn1 -- PS Product13/LConn2
  PS Product8/RConn1 -- PS Product11/LConn2
  PS Product8/LConn2 -- PS Product4/RConn1
  variable CT3/RConn1 -- PS Product8/LConn1
  PS Gain2/LConn1 -- PS Product13/RConn1
  PS Gain1/LConn1 -- PS Product12/RConn1

== system Alpha_Drone_Model/new_drone/Landers1 ==
  Spatial Contact Force{,1..3} (4 alike) : sm_lib/Forces and Torques/Spatial Contact Force  CoefficientOfDynamicFriction=0.3  CoefficientOfStaticFriction=0.5  NormalDamping=5e2  NormalDampingUnits=N/(m/s)  NormalStiffness=3e5  NormalStiffnessUnits=N/m  FrictionalCriticalVelocity=1e-3  FrictionalCriticalVelocityUnits=m/s  ZeroCrossDetectContactStartAndEnd=off  SenseFrictionalForceMagnitude=off  SenseNormalForceMagnitude=off  SenseSeparationDistance=off  NormalTransitionRegionWidth=1e-4  NormalTransitionRegionWidthUnits=m  FrictionType=None
  lander_1_RIGID : Subsystem
  lander_5_RIGID : Subsystem
  lander_6_RIGID : Subsystem
  lander_7_RIGID : Subsystem
  L1 : PMIOPort  Side=Left
  L2 : PMIOPort  Port=2  Side=Left
  L3 : PMIOPort  Port=3  Side=Left
  L4 : PMIOPort  Port=4  Side=Left
  Ground : PMIOPort  Port=5  Side=Right
  connections:
  lander_7_RIGID/LConn1 -- L4/RConn1
  lander_5_RIGID/LConn1 -- L2/RConn1
  lander_1_RIGID/LConn1 -- L1/RConn1
  lander_6_RIGID/LConn1 -- L3/RConn1
  lander_1_RIGID/RConn1 -- Spatial Contact Force/LConn1
  Spatial Contact Force1/LConn1 -- lander_5_RIGID/RConn1
  Spatial Contact Force3/RConn1 -- Spatial Contact Force2/RConn1 -- Spatial Contact Force1/RConn1 -- Spatial Contact Force/RConn1 -- Ground/RConn1
  Spatial Contact Force2/LConn1 -- lander_6_RIGID/RConn1
  Spatial Contact Force3/LConn1 -- lander_7_RIGID/RConn1

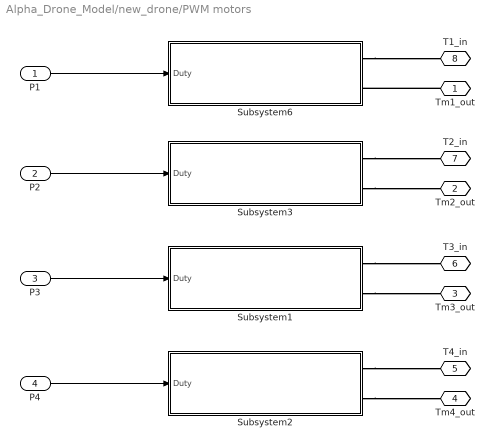
== system Alpha_Drone_Model/new_drone/PWM motors ==
  P1 : Inport
  P2 : Inport  Port=2
  P3 : Inport  Port=3
  P4 : Inport  Port=4
  Subsystem1 : Subsystem
  Subsystem2 : Subsystem
  Subsystem3 : Subsystem
  Subsystem6 : Subsystem
  Tm1_out : PMIOPort  Side=Right
  Tm2_out : PMIOPort  Port=2  Side=Right
  Tm3_out : PMIOPort  Port=3  Side=Right
  Tm4_out : PMIOPort  Port=4  Side=Right
  T4_in : PMIOPort  Port=5  Side=Right
  T3_in : PMIOPort  Port=6  Side=Right
  T2_in : PMIOPort  Port=7  Side=Right
  T1_in : PMIOPort  Port=8  Side=Right
  wires:
  P1/1 -> Subsystem6/1(Duty)
  P3/1 -> Subsystem1/1(Duty)
  P2/1 -> Subsystem3/1(Duty)
  P4/1 -> Subsystem2/1(Duty)
  connections:
  Subsystem2/RConn2 -- Tm4_out/RConn1
  Subsystem6/RConn1 -- T1_in/RConn1
  Subsystem3/RConn2 -- Tm2_out/RConn1
  Subsystem3/RConn1 -- T2_in/RConn1
  Tm1_out/RConn1 -- Subsystem6/RConn2
  Subsystem1/RConn1 -- T3_in/RConn1
  Subsystem1/RConn2 -- Tm3_out/RConn1
  Subsystem2/RConn1 -- T4_in/RConn1

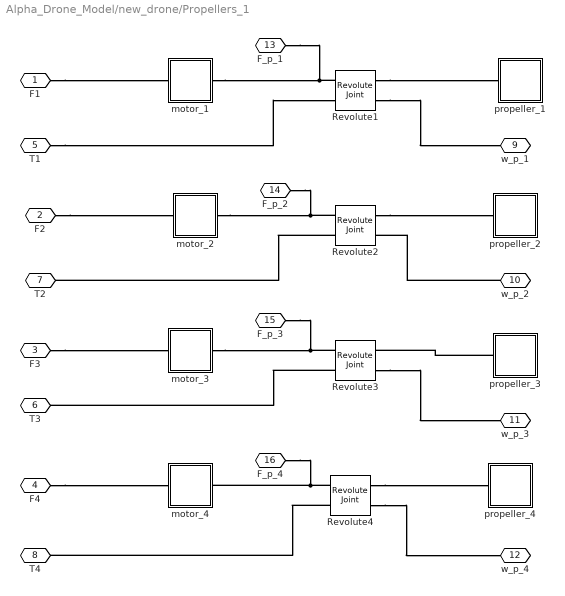
== system Alpha_Drone_Model/new_drone/Propellers_1 ==
  Revolute1 : sm_lib/Joints/Revolute Joint  JointMode=Normal  SenseConstraintForce=off  SenseConstraintForceX=off  SenseConstraintForceY=off  SenseConstraintForceZ=off  SenseConstraintTorque=off  SenseConstraintTorqueX=off  SenseConstraintTorqueY=off  SenseConstraintTorqueZ=off  SenseTotalForce=off  SenseTotalForceX=off  SenseTotalForceY=off  SenseTotalForceZ=off  SenseTotalTorque=off  SenseTotalTorqueX=off  SenseTotalTorqueY=off  SenseTotalTorqueZ=off  CompositeWrenchDir=FollowerOnBase  CompositeWrenchFrame=BaseFrame  EquilibriumPosition=0  EquilibriumPositionUnits=deg  SpringStiffness=0  SpringStiffnessUnits=N*m/deg  DampingCoefficient=0  DampingCoefficientUnits=N*m/(deg/s)  TorqueActuationMode=InputTorque  MotionActuationMode=ComputedMotion  SensePosition=off  SenseVelocity=on  SenseAcceleration=off  SenseTorqueForce=off  SenseLowerLimitTorqueForce=off  SenseUpperLimitTorqueForce=off  LowerLimitSpecify=off  LowerLimitBound=-90  LowerLimitBoundUnits=deg  LowerLimitStiffness=1e4  LowerLimitStiffnessUnits=N*m/deg  LowerLimitDamping=10  LowerLimitDampingUnits=N*m/(deg/s)  LowerLimitTransitionRegionWidth=0.1  LowerLimitTransitionRegionWidthUnits=deg  UpperLimitSpecify=off  UpperLimitBound=90  UpperLimitBoundUnits=deg  UpperLimitStiffness=1e4  UpperLimitStiffnessUnits=N*m/deg  UpperLimitDamping=10  UpperLimitDampingUnits=N*m/(deg/s)  UpperLimitTransitionRegionWidth=0.1  UpperLimitTransitionRegionWidthUnits=deg  PositionTargetSpecify=on  PositionTargetPriority=Low  PositionTargetValue=90  PositionTargetValueUnits=deg  VelocityTargetSpecify=off  VelocityTargetPriority=High  VelocityTargetValue=0  VelocityTargetValueUnits=deg/s
  Revolute2 : sm_lib/Joints/Revolute Joint  JointMode=Normal  SenseConstraintForce=off  SenseConstraintForceX=off  SenseConstraintForceY=off  SenseConstraintForceZ=off  SenseConstraintTorque=off  SenseConstraintTorqueX=off  SenseConstraintTorqueY=off  SenseConstraintTorqueZ=off  SenseTotalForce=off  SenseTotalForceX=off  SenseTotalForceY=off  SenseTotalForceZ=off  SenseTotalTorque=off  SenseTotalTorqueX=off  SenseTotalTorqueY=off  SenseTotalTorqueZ=off  CompositeWrenchDir=FollowerOnBase  CompositeWrenchFrame=BaseFrame  EquilibriumPosition=0  EquilibriumPositionUnits=deg  SpringStiffness=0  SpringStiffnessUnits=N*m/deg  DampingCoefficient=0  DampingCoefficientUnits=N*m/(deg/s)  TorqueActuationMode=InputTorque  MotionActuationMode=ComputedMotion  SensePosition=off  SenseVelocity=on  SenseAcceleration=off  SenseTorqueForce=off  SenseLowerLimitTorqueForce=off  SenseUpperLimitTorqueForce=off  LowerLimitSpecify=off  LowerLimitBound=-90  LowerLimitBoundUnits=deg  LowerLimitStiffness=1e4  LowerLimitStiffnessUnits=N*m/deg  LowerLimitDamping=10  LowerLimitDampingUnits=N*m/(deg/s)  LowerLimitTransitionRegionWidth=0.1  LowerLimitTransitionRegionWidthUnits=deg  UpperLimitSpecify=off  UpperLimitBound=90  UpperLimitBoundUnits=deg  UpperLimitStiffness=1e4  UpperLimitStiffnessUnits=N*m/deg  UpperLimitDamping=10  UpperLimitDampingUnits=N*m/(deg/s)  UpperLimitTransitionRegionWidth=0.1  UpperLimitTransitionRegionWidthUnits=deg  PositionTargetSpecify=on  PositionTargetPriority=Low  PositionTargetValue=0  PositionTargetValueUnits=deg  VelocityTargetSpecify=off  VelocityTargetPriority=High  VelocityTargetValue=0  VelocityTargetValueUnits=deg/s
  Revolute3 : sm_lib/Joints/Revolute Joint  JointMode=Normal  SenseConstraintForce=off  SenseConstraintForceX=off  SenseConstraintForceY=off  SenseConstraintForceZ=off  SenseConstraintTorque=off  SenseConstraintTorqueX=off  SenseConstraintTorqueY=off  SenseConstraintTorqueZ=off  SenseTotalForce=off  SenseTotalForceX=off  SenseTotalForceY=off  SenseTotalForceZ=off  SenseTotalTorque=off  SenseTotalTorqueX=off  SenseTotalTorqueY=off  SenseTotalTorqueZ=off  CompositeWrenchDir=FollowerOnBase  CompositeWrenchFrame=BaseFrame  EquilibriumPosition=0  EquilibriumPositionUnits=deg  SpringStiffness=0  SpringStiffnessUnits=N*m/deg  DampingCoefficient=0  DampingCoefficientUnits=N*m/(deg/s)  TorqueActuationMode=InputTorque  MotionActuationMode=ComputedMotion  SensePosition=off  SenseVelocity=on  SenseAcceleration=off  SenseTorqueForce=off  SenseLowerLimitTorqueForce=off  SenseUpperLimitTorqueForce=off  LowerLimitSpecify=off  LowerLimitBound=-90  LowerLimitBoundUnits=deg  LowerLimitStiffness=1e4  LowerLimitStiffnessUnits=N*m/deg  LowerLimitDamping=10  LowerLimitDampingUnits=N*m/(deg/s)  LowerLimitTransitionRegionWidth=0.1  LowerLimitTransitionRegionWidthUnits=deg  UpperLimitSpecify=off  UpperLimitBound=90  UpperLimitBoundUnits=deg  UpperLimitStiffness=1e4  UpperLimitStiffnessUnits=N*m/deg  UpperLimitDamping=10  UpperLimitDampingUnits=N*m/(deg/s)  UpperLimitTransitionRegionWidth=0.1  UpperLimitTransitionRegionWidthUnits=deg  PositionTargetSpecify=on  PositionTargetPriority=Low  PositionTargetValue=90  PositionTargetValueUnits=deg  VelocityTargetSpecify=off  VelocityTargetPriority=High  VelocityTargetValue=0  VelocityTargetValueUnits=deg/s
  Revolute4 : sm_lib/Joints/Revolute Joint  JointMode=Normal  SenseConstraintForce=off  SenseConstraintForceX=off  SenseConstraintForceY=off  SenseConstraintForceZ=off  SenseConstraintTorque=off  SenseConstraintTorqueX=off  SenseConstraintTorqueY=off  SenseConstraintTorqueZ=off  SenseTotalForce=off  SenseTotalForceX=off  SenseTotalForceY=off  SenseTotalForceZ=off  SenseTotalTorque=off  SenseTotalTorqueX=off  SenseTotalTorqueY=off  SenseTotalTorqueZ=off  CompositeWrenchDir=FollowerOnBase  CompositeWrenchFrame=BaseFrame  EquilibriumPosition=0  EquilibriumPositionUnits=deg  SpringStiffness=0  SpringStiffnessUnits=N*m/deg  DampingCoefficient=0  DampingCoefficientUnits=N*m/(deg/s)  TorqueActuationMode=InputTorque  MotionActuationMode=ComputedMotion  SensePosition=off  SenseVelocity=on  SenseAcceleration=off  SenseTorqueForce=off  SenseLowerLimitTorqueForce=off  SenseUpperLimitTorqueForce=off  LowerLimitSpecify=off  LowerLimitBound=-90  LowerLimitBoundUnits=deg  LowerLimitStiffness=1e4  LowerLimitStiffnessUnits=N*m/deg  LowerLimitDamping=10  LowerLimitDampingUnits=N*m/(deg/s)  LowerLimitTransitionRegionWidth=0.1  LowerLimitTransitionRegionWidthUnits=deg  UpperLimitSpecify=off  UpperLimitBound=90  UpperLimitBoundUnits=deg  UpperLimitStiffness=1e4  UpperLimitStiffnessUnits=N*m/deg  UpperLimitDamping=10  UpperLimitDampingUnits=N*m/(deg/s)  UpperLimitTransitionRegionWidth=0.1  UpperLimitTransitionRegionWidthUnits=deg  PositionTargetSpecify=on  PositionTargetPriority=Low  PositionTargetValue=0  PositionTargetValueUnits=deg  VelocityTargetSpecify=off  VelocityTargetPriority=High  VelocityTargetValue=0  VelocityTargetValueUnits=deg/s
  motor_1 : Subsystem
  motor_2 : Subsystem
  motor_3 : Subsystem
  motor_4 : Subsystem
  propeller_1 : Subsystem
  propeller_2 : Subsystem
  propeller_3 : Subsystem
  propeller_4 : Subsystem
  F1 : PMIOPort  Side=Left
  F2 : PMIOPort  Port=2  Side=Left
  F3 : PMIOPort  Port=3  Side=Left
  F4 : PMIOPort  Port=4  Side=Left
  T1 : PMIOPort  Port=5  Side=Left
  T3 : PMIOPort  Port=6  Side=Left
  T2 : PMIOPort  Port=7  Side=Left
  T4 : PMIOPort  Port=8  Side=Left
  w_p_1 : PMIOPort  Port=9  Side=Right
  w_p_2 : PMIOPort  Port=10  Side=Right
  w_p_3 : PMIOPort  Port=11  Side=Right
  w_p_4 : PMIOPort  Port=12  Side=Right
  F_p_1 : PMIOPort  Port=13  Side=Right
  F_p_2 : PMIOPort  Port=14  Side=Right
  F_p_3 : PMIOPort  Port=15  Side=Right
  F_p_4 : PMIOPort  Port=16  Side=Right
  connections:
  F2/RConn1 -- motor_2/LConn1
  F1/RConn1 -- motor_1/LConn1
  F3/RConn1 -- motor_3/LConn1
  F4/RConn1 -- motor_4/LConn1
  F_p_1/RConn1 -- motor_1/RConn1 -- Revolute1/LConn1
  T1/RConn1 -- Revolute1/LConn2
  Revolute1/RConn2 -- w_p_1/RConn1
  F_p_3/RConn1 -- Revolute3/LConn1 -- motor_3/RConn1
  Revolute3/LConn2 -- T3/RConn1
  Revolute3/RConn2 -- w_p_3/RConn1
  F_p_2/RConn1 -- Revolute2/LConn1 -- motor_2/RConn1
  w_p_2/RConn1 -- Revolute2/RConn2
  F_p_4/RConn1 -- Revolute4/LConn1 -- motor_4/RConn1
  Revolute4/RConn2 -- w_p_4/RConn1
  Revolute2/LConn2 -- T2/RConn1
  Revolute4/LConn2 -- T4/RConn1
  Revolute1/RConn1 -- propeller_1/LConn1
  Revolute2/RConn1 -- propeller_2/LConn1
  propeller_3/LConn1 -- Revolute3/RConn1
  Revolute4/RConn1 -- propeller_4/LConn1

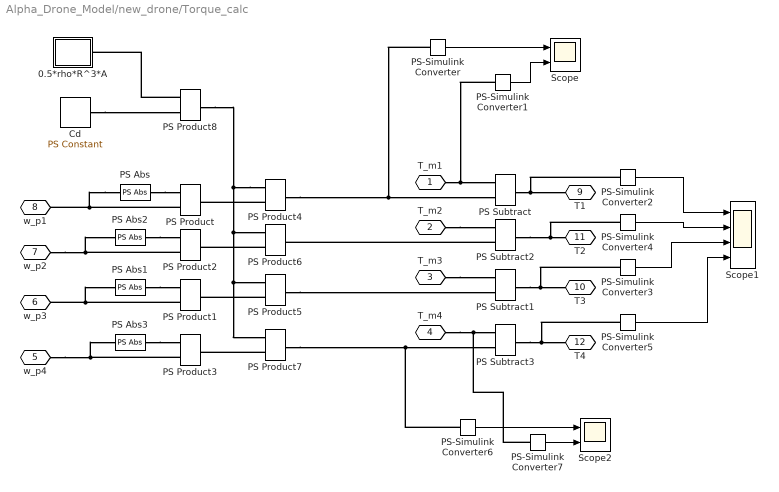
== system Alpha_Drone_Model/new_drone/Torque_calc ==
  0.5*rho*R^3*A : Subsystem
  Cd : fl_lib/Physical Signals/Sources/PS Constant  constant=Cd
  PS Abs{,1..3} (4 alike) : fl_lib/Physical Signals/Nonlinear Operators/PS Abs
      settings: SourceProductBaseCode=SS  InternalSimscapePortConfiguration="{\"Bottom\":[],\"Left\":[{\"id\":\"I\",\"label\":\"\",\"type\":\"input\"}],\"Right\":[{\"id\":\"O\",\"label\":\"\",\"type\":\"output\"}],\"Top\":[]}"
  PS Product{,1..8} (9 alike) : fl_lib/Physical Signals/Functions/PS Product
  PS Subtract{,1..3} (4 alike) : fl_lib/Physical Signals/Functions/PS Subtract
  PS-Simulink Converter{,1..7} (8 alike) : nesl_utility/PS-Simulink Converter  PhysicalDomain=network_engine_domain  SubClassName=ps_output  LeftPortType=input  RightPortType=output  PseudoPeriodic=off  Frequencies=[]  Unit=inherit  AffineConversion=off
  Scope : Scope  NumInputPorts=2
  Scope1 : Scope  NumInputPorts=4
  Scope2 : Scope  NumInputPorts=2
  T_m1 : PMIOPort  Side=Left
  T_m2 : PMIOPort  Port=2  Side=Left
  T_m3 : PMIOPort  Port=3  Side=Left
  T_m4 : PMIOPort  Port=4  Side=Left
  w_p4 : PMIOPort  Port=5  Side=Right
  w_p3 : PMIOPort  Port=6  Side=Right
  w_p2 : PMIOPort  Port=7  Side=Right
  w_p1 : PMIOPort  Port=8  Side=Right
  T1 : PMIOPort  Port=9  Side=Right
  T3 : PMIOPort  Port=10  Side=Right
  T2 : PMIOPort  Port=11  Side=Right
  T4 : PMIOPort  Port=12  Side=Right
  wires:
  PS-Simulink Converter/1 -> Scope/1
  PS-Simulink Converter1/1 -> Scope/2
  PS-Simulink Converter2/1 -> Scope1/1
  PS-Simulink Converter5/1 -> Scope1/4
  PS-Simulink Converter7/1 -> Scope2/2
  PS-Simulink Converter6/1 -> Scope2/1
  PS-Simulink Converter4/1 -> Scope1/2
  PS-Simulink Converter3/1 -> Scope1/3
  connections:
  PS Abs/RConn1 -- PS Product/LConn1
  PS Product4/LConn2 -- PS Product/RConn1
  PS Product1/LConn2 -- w_p3/RConn1 -- PS Abs1/LConn1
  PS Product5/LConn2 -- PS Product1/RConn1
  PS Abs2/RConn1 -- PS Product2/LConn1
  PS Product3/LConn2 -- w_p4/RConn1 -- PS Abs3/LConn1
  PS Product7/LConn2 -- PS Product3/RConn1
  PS Product6/LConn2 -- PS Product2/RConn1
  PS Subtract/RConn1 -- PS-Simulink Converter2/LConn1 -- T1/RConn1
  PS Subtract2/RConn1 -- PS-Simulink Converter4/LConn1 -- T2/RConn1
  PS Subtract1/RConn1 -- PS-Simulink Converter3/LConn1 -- T3/RConn1
  PS Subtract3/RConn1 -- PS-Simulink Converter5/LConn1 -- T4/RConn1
  T_m1/RConn1 -- PS-Simulink Converter1/LConn1 -- PS Subtract/LConn1
  PS Product4/RConn1 -- PS-Simulink Converter/LConn1 -- PS Subtract/LConn2
  PS Product5/RConn1 -- PS Subtract1/LConn2
  PS Subtract2/LConn2 -- PS Product6/RConn1
  PS Product7/RConn1 -- PS-Simulink Converter6/LConn1 -- PS Subtract3/LConn2
  T_m2/RConn1 -- PS Subtract2/LConn1
  T_m3/RConn1 -- PS Subtract1/LConn1
  T_m4/RConn1 -- PS-Simulink Converter7/LConn1 -- PS Subtract3/LConn1
  PS Abs/LConn1 -- PS Product/LConn2 -- w_p1/RConn1
  PS Abs1/RConn1 -- PS Product1/LConn1
  w_p2/RConn1 -- PS Product2/LConn2 -- PS Abs2/LConn1
  PS Abs3/RConn1 -- PS Product3/LConn1
  PS Product8/LConn1 -- 0.5*rho*R^3*A/RConn1
  Cd/RConn1 -- PS Product8/LConn2
  PS Product4/LConn1 -- PS Product8/RConn1 -- PS Product6/LConn1 -- PS Product7/LConn1 -- PS Product5/LConn1

== system Alpha_Drone_Model/new_drone/Drone/Subsystem ==
  drone_pillar_test_2_1_RIGID : Subsystem
  drone_pillar_test_2_2_RIGID : Subsystem
  drone_pillar_test_2_3_RIGID : Subsystem
  drone_pillar_test_2_4_RIGID : Subsystem
  F : PMIOPort  Side=Left
  F1 : PMIOPort  Port=2  Side=Left
  F3 : PMIOPort  Port=3  Side=Left
  F4 : PMIOPort  Port=4  Side=Left
  connections:
  drone_pillar_test_2_3_RIGID/LConn1 -- F1/RConn1
  drone_pillar_test_2_2_RIGID/LConn1 -- F3/RConn1
  F/RConn1 -- drone_pillar_test_2_4_RIGID/LConn1
  F4/RConn1 -- drone_pillar_test_2_1_RIGID/LConn1

== system Alpha_Drone_Model/new_drone/Drone/Subsystem1 ==
  drone_antenna_holder_test_1_RIGID : Subsystem
  drone_antenna_test_1_RIGID : Subsystem
  drone_camera_and_proximity_sensor_weight_1_RIGID : Subsystem
  drone_camera_wall_test_1_RIGID : Subsystem
  drone_camera_wall_test_2_RIGID : Subsystem
  drone_chip_2_test_1_RIGID : Subsystem
  drone_fc_test_1_RIGID : Subsystem
  F1 : PMIOPort  Side=Left
  F : PMIOPort  Port=2  Side=Left
  F2 : PMIOPort  Port=3  Side=Left
  F3 : PMIOPort  Port=4  Side=Left
  F4 : PMIOPort  Port=5  Side=Left
  connections:
  drone_antenna_holder_test_1_RIGID/RConn1 -- drone_antenna_test_1_RIGID/LConn1
  F3/RConn1 -- drone_fc_test_1_RIGID/LConn1
  F/RConn1 -- drone_camera_wall_test_1_RIGID/LConn1
  drone_camera_wall_test_1_RIGID/RConn1 -- drone_camera_and_proximity_sensor_weight_1_RIGID/LConn1
  F4/RConn1 -- drone_chip_2_test_1_RIGID/LConn1
  F2/RConn1 -- drone_camera_wall_test_2_RIGID/LConn1
  drone_antenna_holder_test_1_RIGID/LConn1 -- F1/RConn1

== system Alpha_Drone_Model/new_drone/Drone/Subsystem2 ==
  drone_battery_cell_1_1_RIGID : Subsystem
  drone_battery_cell_1_2_RIGID : Subsystem
  drone_top_test_3_1_RIGID : Subsystem
  F : PMIOPort  Side=Left
  connections:
  drone_battery_cell_1_1_RIGID/LConn1 -- drone_battery_cell_1_2_RIGID/LConn1
  drone_battery_cell_1_1_RIGID/LConn2 -- drone_top_test_3_1_RIGID/RConn1
  drone_top_test_3_1_RIGID/LConn1 -- F/RConn1
